simulink model "bouncing_ball"  (R2017a)
settings: Solver=FixedStepAuto  StartTime=0.0  StopTime=10  FixedStep=0.1  RelTol=1e-3
settings Model: Creator=xiaodong  LastModifiedBy=xiaodong
settings DataIOCC: SaveFormat=Array  SaveOutput=off  SaveTime=off

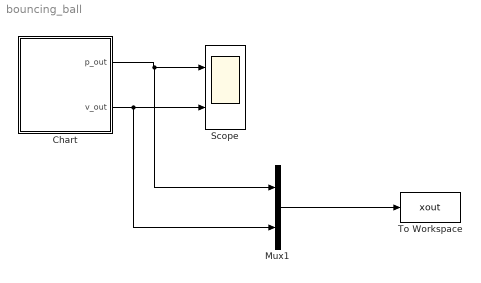
== system bouncing_ball ==
  Chart : Stateflow chart  TreatAsAtomicUnit=on
  Mux1 : Mux  Inputs=2
  Scope : Scope  NumInputPorts=2
  To Workspace : ToWorkspace  VariableName=xout  SampleTime=0.1
  wires:
  Chart/1(p_out) -> Mux1/1, Scope/1
  Chart/2(v_out) -> Mux1/2, Scope/2
  Mux1/1 -> To Workspace/1

== stateflow chart bouncing_ball/Chart ==
  settings: updateMethod=CONTINUOUS
  state Falling
    du:
    p_dot= v;
    v_dot = -9.81;
    p_out = p;
    v_out=v;
  (default) -> Falling : {p =16; v = 15;}
  Falling -> Falling : [p<=0 && v<0]{p=0; v=-0.8.*v}
  data: p local; v local; p_out output; v_out output
  data p settings: updateMethod=SF_CONTINUOUS_TIME_DATA
  data v settings: updateMethod=SF_CONTINUOUS_TIME_DATA
